simulink model "sideslip_estimation"  (R2017b)
settings: Solver=VariableStepAuto  StartTime=0.0  StopTime=10.0  RelTol=1e-3
settings Model: Creator=Dell  LastModifiedBy=Dell

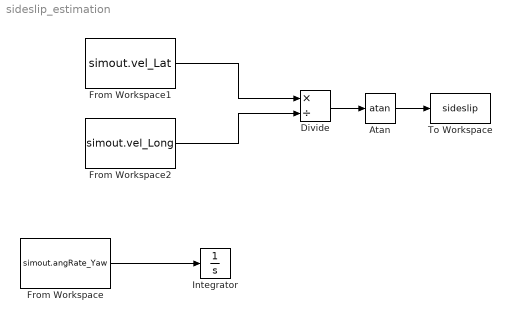
== system sideslip_estimation ==
  Atan : Trigonometry  Operator=atan
  Divide : Product  Inputs=*/
  From Workspace : FromWorkspace  VariableName=simout.angRate_Yaw  SampleTime=0
  From Workspace1 : FromWorkspace  VariableName=simout.vel_Lat  SampleTime=0
  From Workspace2 : FromWorkspace  VariableName=simout.vel_Long  SampleTime=0
  Integrator : Integrator
  To Workspace : ToWorkspace  VariableName=sideslip  SaveFormat=Timeseries  SampleTime=-1
  wires:
  From Workspace/1 -> Integrator/1
  From Workspace1/1 -> Divide/1
  From Workspace2/1 -> Divide/2
  Divide/1 -> Atan/1
  Atan/1 -> To Workspace/1
